simulink model "simulation_X4_PIDout"  (Simulink 8.8)
settings: Solver=ode45  StartTime=0.0  StopTime=10  MaxStep=0.01  RelTol=1e-6  EnableMultiTasking=on
values from neighbouring files (symbols this model uses):
  Ixx = 0.0294853730990492 * 1    (= 0.029485373099)    [main_tune_gain.m]
  Ixz = 0.0000    (= 0)    [main_tune_gain.m]
  Iyy = 0.0636259128602231 * 1    (= 0.0636259128602)    [main_tune_gain.m]
  Izz = 0.0809362287249525 * 1    (= 0.080936228725)    [main_tune_gain.m]
  omega_n_m = 30    [main_tune_gain.m]
  omega_trans_x_out = 0.1    [main_tune_gain.m]
  omega_trans_y_out = 0.1    [main_tune_gain.m]
  omega_trans_z_out = 0.5    [main_tune_gain.m]
  XD = 1.4    [main_tune_gain.m]
  XI = 0.1    [main_tune_gain.m]
  xi_m = 0.707    [main_tune_gain.m]
  XP = 0.1    [main_tune_gain.m]
  YD = 0.4    [main_tune_gain.m]
  YI = 0.1    [main_tune_gain.m]
  YP = 0.8    [main_tune_gain.m]
  ZD = 2    [main_tune_gain.m]
  ZI = 0.02    [main_tune_gain.m]
  ZP = 1    [main_tune_gain.m]
undefined symbols (not defined in the file or in its folder): attitude_control_allocation, compute_com_position
settings Model: SuppressorTable=22 serialization::archive 11 0 3 0 0 0 11 0  Creator=t  LastModifiedBy=root
settings OptimizationCC: ExpressionDepthLimit=2147483647  InitFltsAndDblsToZero=on
settings DebuggingCC: SaveWithParameterizedLinksMsg=none  SolverPrmCheckMsg=warning
settings GRTTargetCC: TargetFcnLib=ansi_tfl_tmw.mat

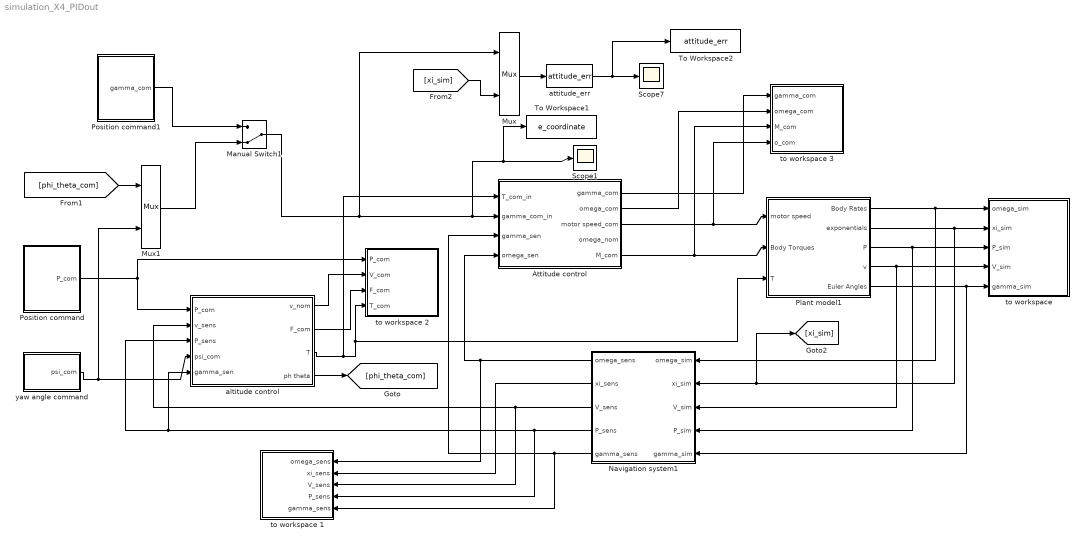
== system simulation_X4_PIDout ==
  Attitude control : Subsystem
  Manual Switch1 : ManualSwitch  CurrentSetting=0
  Mux : Mux  Inputs=2
  Mux1 : Mux  Inputs=2
  Navigation system1 : Subsystem
  Plant model1 : Subsystem
  Position command : Subsystem
  Position command1 : Subsystem
  Scope1 : Scope
  Scope7 : Scope
  To Workspace1 : ToWorkspace  VariableName=e_coordinate  SampleTime=-1
  To Workspace2 : ToWorkspace  VariableName=attitude_err  SampleTime=-1
  altitude control : Subsystem
  attitude_err : MATLABFcn  MATLABFcn=attitude_err
  to workspace : Subsystem
      settings: AttributesFormatString=%<AncestorBlock>
  to workspace 1 : Subsystem
      settings: AttributesFormatString=%<AncestorBlock>
  to workspace 2 : Subsystem
      settings: AttributesFormatString=%<AncestorBlock>
  to workspace 3 : Subsystem
      settings: AttributesFormatString=%<AncestorBlock>
  yaw angle command : Subsystem
  wires:
  Attitude control/3(motor speed_com) -> Plant model1/1(motor speed), to workspace 3/4(o_com)
  Navigation system1/1(omega_sens) -> Attitude control/4(omega_sen), to workspace 1/1(omega_sens)
  Navigation system1/2(xi_sens) -> to workspace 1/2(xi_sens)
  Navigation system1/3(V_sens) -> to workspace 1/3(V_sens), altitude control/2(v_sens)
  Navigation system1/4(P_sens) -> to workspace 1/4(P_sens), altitude control/3(P_sens), altitude control/5(gamma_sen)
  Attitude control/1(gamma_com) -> to workspace 3/1(gamma_com)
  Attitude control/2(omega_com) -> to workspace 3/2(omega_com)
  Attitude control/5(M_com) -> to workspace 3/3(M_com), Plant model1/2(Body Torques)
  Position command/1(P_com) -> altitude control/1(P_com), to workspace 2/1(P_com)
  Plant model1/1(Body Rates) -> to workspace/1(omega_sim), Navigation system1/1(omega_sim)
  Plant model1/2(exponentials) -> to workspace/2(xi_sim), Navigation system1/2(xi_sim), [xi_sim]
  Mux/1 -> attitude_err/1
  attitude_err/1 -> Scope7/1, To Workspace2/1
  altitude control/1(v_nom) -> to workspace 2/2(V_com)
  yaw angle command/1(psi_com) -> Mux1/2, altitude control/4(psi_com)
  Plant model1/3(P) -> to workspace/3(P_sim), Navigation system1/4(P_sim)
  Plant model1/4(v) -> to workspace/4(V_sim), Navigation system1/3(V_sim)
  Plant model1/5(Euler Angles) -> to workspace/5(gamma_sim), Navigation system1/5(gamma_sim)
  Navigation system1/5(gamma_sens) -> to workspace 1/5(gamma_sens), Attitude control/3(gamma_sen)
  [xi_sim] -> Mux/2
  altitude control/2(F_com) -> to workspace 2/3(F_com)
  altitude control/4(ph theta) -> [phi_theta_com]
  [phi_theta_com] -> Mux1/1
  altitude control/3(T) -> Plant model1/3(T), to workspace 2/4(T_com), Attitude control/1(T_com_in)
  Position command1/1(gamma_com) -> Manual Switch1/1
  Manual Switch1/1 -> Attitude control/2(gamma_com_in), Scope1/1, To Workspace1/1, Mux/1
  Mux1/1 -> Manual Switch1/2

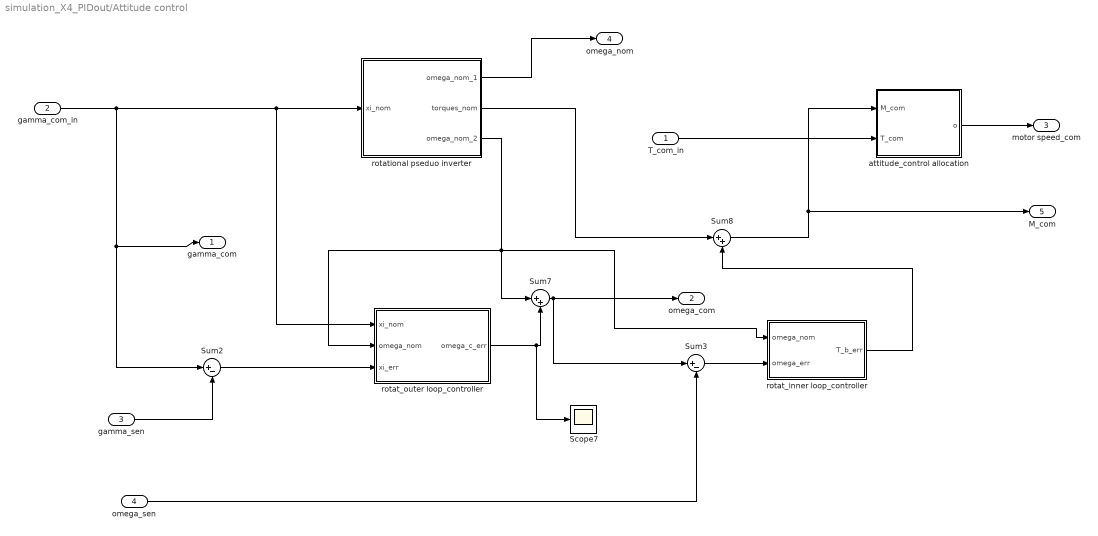
== system simulation_X4_PIDout/Attitude control ==
  T_com_in : Inport
  gamma_com_in : Inport  Port=2
  gamma_sen : Inport  Port=3
  omega_sen : Inport  Port=4
  Scope7 : Scope
  Sum2 : Sum  Inputs=|+-
  Sum3 : Sum  Inputs=|+-
  Sum7 : Sum  Inputs=|++
  Sum8 : Sum  Inputs=|++
  attitude_control allocation : Subsystem
  rotat_inner loop_controller : Subsystem
  rotat_outer loop_controller : Subsystem
  rotational pseduo inverter : Subsystem
  gamma_com : Outport
  omega_com : Outport  Port=2
  motor speed_com : Outport  Port=3
  omega_nom : Outport  Port=4
  M_com : Outport  Port=5
  wires:
  gamma_com_in/1 -> rotational pseduo inverter/1(xi_nom), rotat_outer loop_controller/1(xi_nom), Sum2/1, gamma_com/1
  Sum2/1 -> rotat_outer loop_controller/3(xi_err)
  rotational pseduo inverter/3(omega_nom_2) -> Sum7/1, rotat_outer loop_controller/2(omega_nom), rotat_inner loop_controller/1(omega_nom)
  Sum7/1 -> Sum3/1, omega_com/1
  Sum3/1 -> rotat_inner loop_controller/2(omega_err)
  rotational pseduo inverter/2(torques_nom) -> Sum8/1
  Sum8/1 -> attitude_control allocation/1(M_com), M_com/1
  gamma_sen/1 -> Sum2/2
  omega_sen/1 -> Sum3/2
  rotat_inner loop_controller/1(T_b_err) -> Sum8/2
  rotational pseduo inverter/1(omega_nom_1) -> omega_nom/1
  attitude_control allocation/1(o) -> motor speed_com/1
  T_com_in/1 -> attitude_control allocation/2(T_com)
  rotat_outer loop_controller/1(omega_c_err) -> Sum7/2, Scope7/1

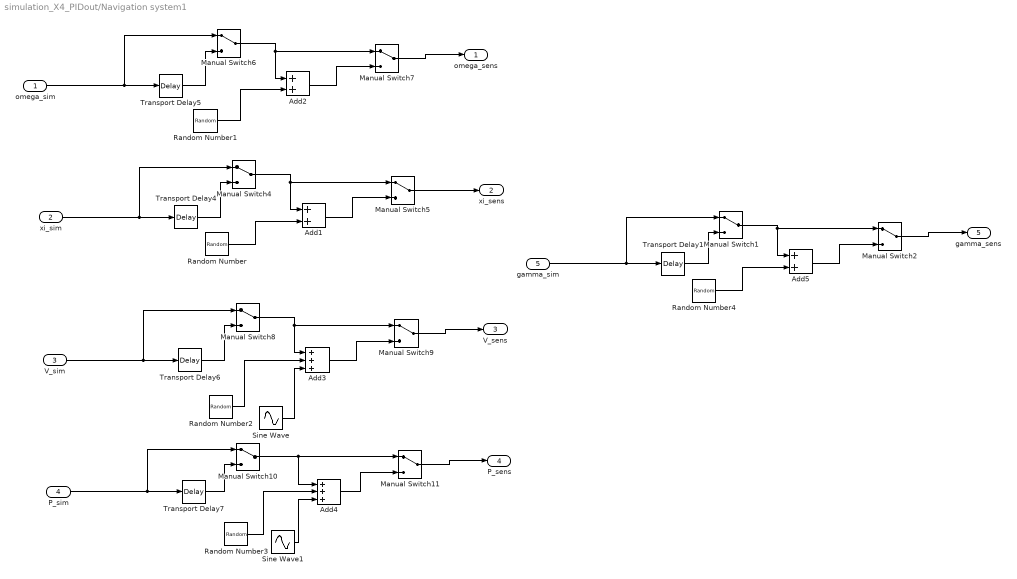
== system simulation_X4_PIDout/Navigation system1 ==
  omega_sim : Inport
  xi_sim : Inport  Port=2
  V_sim : Inport  Port=3
  P_sim : Inport  Port=4
  gamma_sim : Inport  Port=5
  Add1 : Sum
  Add2 : Sum
  Add3 : Sum  Inputs=+++
  Add4 : Sum  Inputs=+++
  Add5 : Sum
  Manual Switch{1..2,4..11} (10 alike) : ManualSwitch
  Random Number : RandomNumber  Variance=0.000025  SampleTime=0
  Random Number1 : RandomNumber  Variance=0.001  SampleTime=0
  Random Number2 : RandomNumber  Variance=0.001  SampleTime=0
  Random Number3 : RandomNumber  Variance=0.001  SampleTime=0
  Random Number4 : RandomNumber  Variance=0.000025  SampleTime=0
  Sine Wave : Sin  Amplitude=0.2  SampleTime=0
  Sine Wave1 : Sin  Amplitude=1.5  SampleTime=0
  Transport Delay1 : TransportDelay  DelayTime=0.02
  Transport Delay4 : TransportDelay  DelayTime=0.02
  Transport Delay5 : TransportDelay  DelayTime=0.02
  Transport Delay6 : TransportDelay  DelayTime=0.4
  Transport Delay7 : TransportDelay  DelayTime=0.4
  omega_sens : Outport
  xi_sens : Outport  Port=2
  V_sens : Outport  Port=3
  P_sens : Outport  Port=4
  gamma_sens : Outport  Port=5
  wires:
  xi_sim/1 -> Transport Delay4/1, Manual Switch4/1
  Manual Switch4/1 -> Add1/1, Manual Switch5/1
  Transport Delay4/1 -> Manual Switch4/2
  Manual Switch5/1 -> xi_sens/1
  Random Number/1 -> Add1/2
  Add1/1 -> Manual Switch5/2
  omega_sim/1 -> Transport Delay5/1, Manual Switch6/1
  Manual Switch6/1 -> Add2/1, Manual Switch7/1
  Transport Delay5/1 -> Manual Switch6/2
  Manual Switch7/1 -> omega_sens/1
  Random Number1/1 -> Add2/2
  Add2/1 -> Manual Switch7/2
  V_sim/1 -> Transport Delay6/1, Manual Switch8/1
  Manual Switch8/1 -> Add3/1, Manual Switch9/1
  Transport Delay6/1 -> Manual Switch8/2
  Manual Switch9/1 -> V_sens/1
  Random Number2/1 -> Add3/2
  Add3/1 -> Manual Switch9/2
  P_sim/1 -> Transport Delay7/1, Manual Switch10/1
  Manual Switch10/1 -> Add4/1, Manual Switch11/1
  Transport Delay7/1 -> Manual Switch10/2
  Manual Switch11/1 -> P_sens/1
  Random Number3/1 -> Add4/2
  Add4/1 -> Manual Switch11/2
  gamma_sim/1 -> Transport Delay1/1, Manual Switch1/1
  Manual Switch1/1 -> Add5/1, Manual Switch2/1
  Transport Delay1/1 -> Manual Switch1/2
  Manual Switch2/1 -> gamma_sens/1
  Random Number4/1 -> Add5/2
  Add5/1 -> Manual Switch2/2
  Sine Wave/1 -> Add3/3
  Sine Wave1/1 -> Add4/3

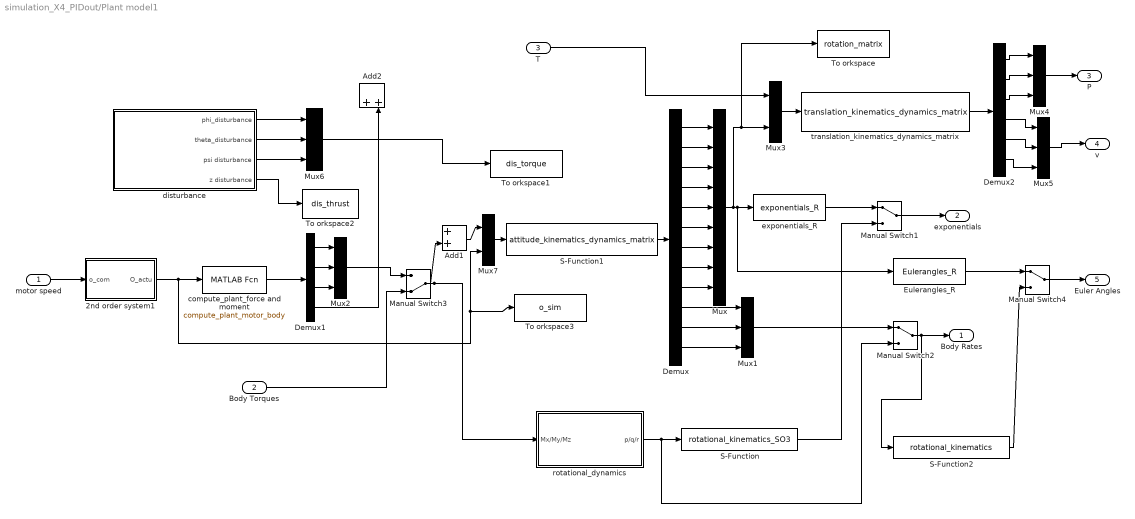
== system simulation_X4_PIDout/Plant model1 ==
  motor speed : Inport
  Body Torques : Inport  Port=2
  T : Inport  Port=3
  2nd order system1 : Subsystem
  Add1 : Sum
  Add2 : Sum
  Demux : Demux  Outputs=12
  Demux1 : Demux
  Demux2 : Demux  Outputs=6
  Eulerangles_R : MATLABFcn  MATLABFcn=Eulerangles_R  OutputDimensions=3
  Manual Switch1 : ManualSwitch
  Manual Switch2 : ManualSwitch
  Manual Switch3 : ManualSwitch  CurrentSetting=0
  Manual Switch4 : ManualSwitch
  Mux : Mux  Inputs=9
  Mux{1..2,4..6} (5 alike) : Mux  Inputs=3
  Mux3 : Mux  Inputs=2
  Mux7 : Mux  Inputs=2
  S-Function : S-Function  FunctionName=rotational_kinematics_SO3  SFunctionDeploymentMode=off  EnableBusSupport=off
  S-Function1 : S-Function  FunctionName=attitude_kinematics_dynamics_matrix  SFunctionDeploymentMode=off  EnableBusSupport=off
  S-Function2 : S-Function  FunctionName=rotational_kinematics  SFunctionDeploymentMode=off  EnableBusSupport=off
  To orkspace : ToWorkspace  VariableName=rotation_matrix  SampleTime=-1
  To orkspace1 : ToWorkspace  VariableName=dis_torque  SampleTime=-1
  To orkspace2 : ToWorkspace  VariableName=dis_thrust  SampleTime=-1
  To orkspace3 : ToWorkspace  VariableName=o_sim  SampleTime=-1
  compute_plant_force and moment : MATLABFcn  MATLABFcn=compute_plant_motor_body
  disturbance : Subsystem
  exponentials_R : MATLABFcn  MATLABFcn=exponentials_R  OutputDimensions=3
  rotational_dynamics : Subsystem
  translation_kinematics_dynamics_matrix : S-Function  FunctionName=translation_kinematics_dynamics_matrix  SFunctionDeploymentMode=off  EnableBusSupport=off
  Body Rates : Outport
  exponentials : Outport  Port=2
  P : Outport  Port=3
  v : Outport  Port=4
  Euler Angles : Outport  Port=5
  wires:
  rotational_dynamics/1(p/q/r) -> S-Function/1, Manual Switch2/2
  S-Function1/1 -> Demux/1
  Demux/1 -> Mux/1
  Demux/2 -> Mux/2
  Demux/3 -> Mux/3
  Demux/4 -> Mux/4
  Demux/5 -> Mux/5
  Demux/6 -> Mux/6
  Demux/7 -> Mux/7
  Demux/8 -> Mux/8
  Demux/9 -> Mux/9
  Demux/10 -> Mux1/1
  Demux/11 -> Mux1/2
  Demux/12 -> Mux1/3
  Mux/1 -> exponentials_R/1, Eulerangles_R/1, Mux3/2, To orkspace/1
  exponentials_R/1 -> Manual Switch1/1
  Mux1/1 -> Manual Switch2/1
  S-Function/1 -> Manual Switch1/2
  Manual Switch1/1 -> exponentials/1
  Manual Switch2/1 -> Body Rates/1, S-Function2/1
  motor speed/1 -> 2nd order system1/1(o_com)
  compute_plant_force and moment/1 -> Demux1/1
  Demux1/1 -> Mux2/1
  Demux1/2 -> Mux2/2
  Demux1/3 -> Mux2/3
  Mux2/1 -> Manual Switch3/1
  Manual Switch3/1 -> rotational_dynamics/1(Mx/My/Mz), Add1/2
  Body Torques/1 -> Manual Switch3/2
  Mux3/1 -> translation_kinematics_dynamics_matrix/1
  translation_kinematics_dynamics_matrix/1 -> Demux2/1
  Demux2/1 -> Mux4/1
  Demux2/2 -> Mux4/2
  Demux2/3 -> Mux4/3
  Demux2/4 -> Mux5/1
  Demux2/5 -> Mux5/2
  Demux2/6 -> Mux5/3
  Mux4/1 -> P/1
  Mux5/1 -> v/1
  Eulerangles_R/1 -> Manual Switch4/1
  S-Function2/1 -> Manual Switch4/2
  Manual Switch4/1 -> Euler Angles/1
  disturbance/1(phi_disturbance) -> Mux6/1
  disturbance/2(theta_disturbance) -> Mux6/2
  disturbance/3(psi disturbance) -> Mux6/3
  Mux6/1 -> To orkspace1/1
  disturbance/4(z disturbance) -> To orkspace2/1
  Demux1/4 -> Add2/2
  2nd order system1/1(O_actu) -> compute_plant_force and moment/1, Mux7/2, To orkspace3/1
  Mux7/1 -> S-Function1/1
  Add1/1 -> Mux7/1
  T/1 -> Mux3/1

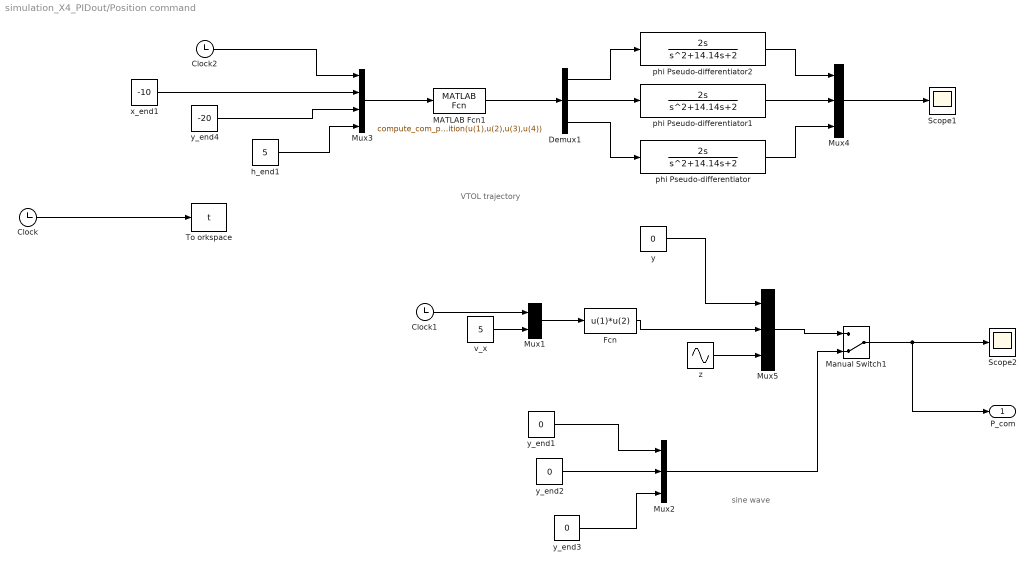
== system simulation_X4_PIDout/Position command ==
  note: VTOL trajectory
  note: sine wave
  Clock : Clock
  Clock1 : Clock
  Clock2 : Clock
  Demux1 : Demux  Outputs=3
  Fcn : Fcn  Expr=u(1)*u(2)
  MATLAB Fcn1 : MATLABFcn  MATLABFcn=compute_com_position(u(1),u(2),u(3),u(4))
  Manual Switch1 : ManualSwitch  CurrentSetting=0
  Mux1 : Mux  Inputs=2
  Mux2 : Mux  Inputs=3
  Mux3 : Mux
  Mux4 : Mux  Inputs=3
  Mux5 : Mux  Inputs=3
  Scope1 : Scope
  Scope2 : Scope
  To orkspace : ToWorkspace  VariableName=t  SampleTime=-1
  h_end1 : Constant  Value=5
  phi Pseudo-differentiator : TransferFcn  Numerator=[2 0]  Denominator=[1 14.14 2]
  phi Pseudo-differentiator1 : TransferFcn  Numerator=[2 0]  Denominator=[1 14.14 2]
  phi Pseudo-differentiator2 : TransferFcn  Numerator=[2 0]  Denominator=[1 14.14 2]
  v_x : Constant  Value=5
  x_end1 : Constant  Value=-10
  y : Constant  Value=0
  y_end1 : Constant  Value=0
  y_end2 : Constant  Value=0
  y_end3 : Constant  Value=0
  y_end4 : Constant  Value=-20
  z : Sin  Frequency=0.5  SampleTime=0
  P_com : Outport
  wires:
  y_end1/1 -> Mux2/1
  y_end2/1 -> Mux2/2
  y_end3/1 -> Mux2/3
  Mux3/1 -> MATLAB Fcn1/1
  Clock2/1 -> Mux3/1
  x_end1/1 -> Mux3/2
  y_end4/1 -> Mux3/3
  h_end1/1 -> Mux3/4
  Demux1/1 -> phi Pseudo-differentiator2/1
  Demux1/2 -> phi Pseudo-differentiator1/1
  Demux1/3 -> phi Pseudo-differentiator/1
  phi Pseudo-differentiator2/1 -> Mux4/1
  phi Pseudo-differentiator1/1 -> Mux4/2
  phi Pseudo-differentiator/1 -> Mux4/3
  MATLAB Fcn1/1 -> Demux1/1
  Mux4/1 -> Scope1/1
  Mux1/1 -> Fcn/1
  Clock1/1 -> Mux1/1
  v_x/1 -> Mux1/2
  Fcn/1 -> Mux5/2
  y/1 -> Mux5/1
  z/1 -> Mux5/3
  Clock/1 -> To orkspace/1
  Mux5/1 -> Manual Switch1/1
  Manual Switch1/1 -> Scope2/1, P_com/1
  Mux2/1 -> Manual Switch1/2

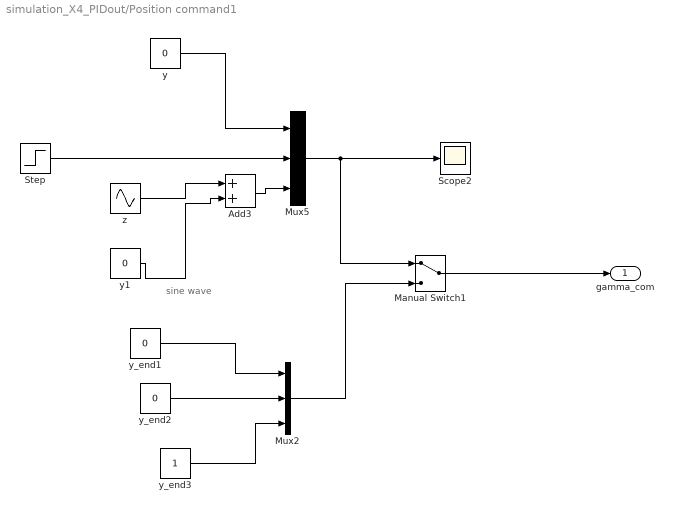
== system simulation_X4_PIDout/Position command1 ==
  note: sine wave
  Add3 : Sum
  Manual Switch1 : ManualSwitch
  Mux2 : Mux  Inputs=3
  Mux5 : Mux  Inputs=3
  Scope2 : Scope
  Step : Step  Time=2  After=0.1  SampleTime=0
  y : Constant  Value=0
  y1 : Constant  Value=0
  y_end1 : Constant  Value=0
  y_end2 : Constant  Value=0
  y_end3 : Constant
  z : Sin  Amplitude=0.1  Frequency=0.5  SampleTime=0
  gamma_com : Outport
  wires:
  y_end1/1 -> Mux2/1
  y_end2/1 -> Mux2/2
  y_end3/1 -> Mux2/3
  Mux5/1 -> Scope2/1, Manual Switch1/1
  y/1 -> Mux5/1
  Mux2/1 -> Manual Switch1/2
  Manual Switch1/1 -> gamma_com/1
  Step/1 -> Mux5/2
  z/1 -> Add3/1
  Add3/1 -> Mux5/3
  y1/1 -> Add3/2

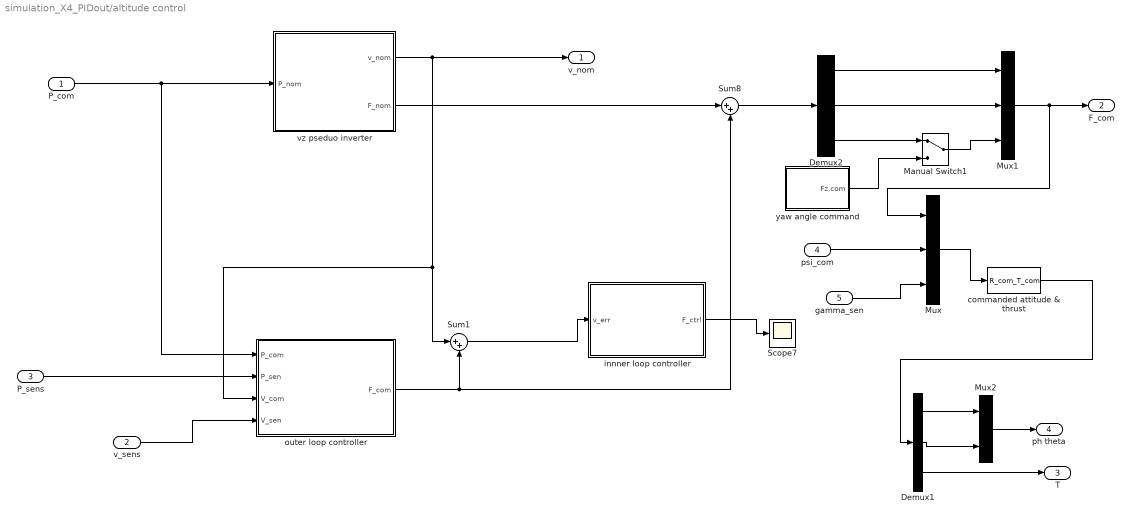
== system simulation_X4_PIDout/altitude control ==
  P_com : Inport
  v_sens : Inport  Port=2
  P_sens : Inport  Port=3
  psi_com : Inport  Port=4
  gamma_sen : Inport  Port=5
  Demux1 : Demux  Outputs=3
  Demux2 : Demux  Outputs=3
  Manual Switch1 : ManualSwitch
  Mux : Mux  Inputs=3
  Mux1 : Mux  Inputs=3
  Mux2 : Mux  Inputs=2
  Scope7 : Scope
  Sum1 : Sum  Inputs=|++
  Sum8 : Sum  Inputs=|++
  commanded attitude & thrust : MATLABFcn  MATLABFcn=R_com_T_com
  innner loop controller : Subsystem
  outer loop controller : Subsystem
  vz pseduo inverter : Subsystem
  yaw angle command : Subsystem
  v_nom : Outport
  F_com : Outport  Port=2
  T : Outport  Port=3
  ph theta : Outport  Port=4
  wires:
  P_com/1 -> vz pseduo inverter/1(P_nom), outer loop controller/1(P_com)
  innner loop controller/1(F_ctrl) -> Scope7/1
  vz pseduo inverter/2(F_nom) -> Sum8/1
  P_sens/1 -> outer loop controller/2(P_sen)
  vz pseduo inverter/1(v_nom) -> v_nom/1, Sum1/1, outer loop controller/3(V_com)
  outer loop controller/1(F_com) -> Sum1/2, Sum8/2
  Sum1/1 -> innner loop controller/1(v_err)
  psi_com/1 -> Mux/2
  Mux/1 -> commanded attitude & thrust/1
  Demux1/1 -> Mux2/1
  Demux1/2 -> Mux2/2
  commanded attitude & thrust/1 -> Demux1/1
  Mux2/1 -> ph theta/1
  Demux1/3 -> T/1
  Sum8/1 -> Demux2/1
  Demux2/3 -> Manual Switch1/1
  Demux2/1 -> Mux1/1
  Demux2/2 -> Mux1/2
  Manual Switch1/1 -> Mux1/3
  Mux1/1 -> F_com/1, Mux/1
  yaw angle command/1(Fz,com) -> Manual Switch1/2
  v_sens/1 -> outer loop controller/4(V_sen)
  gamma_sen/1 -> Mux/3

== system simulation_X4_PIDout/to workspace ==
  omega_sim : Inport
  xi_sim : Inport  Port=2
  P_sim : Inport  Port=3
  V_sim : Inport  Port=4
  gamma_sim : Inport  Port=5
  To Workspace1 : ToWorkspace  VariableName=gamma_sim  SampleTime=-1
  To Workspace2 : ToWorkspace  VariableName=V_sim  SampleTime=-1
  To Workspace3 : ToWorkspace  VariableName=P_sim  SampleTime=-1
  To Workspace4 : ToWorkspace  VariableName=xi_sim  SampleTime=-1
  To orkspace : ToWorkspace  VariableName=omega_sim  SampleTime=-1
  wires:
  omega_sim/1 -> To orkspace/1
  V_sim/1 -> To Workspace2/1
  P_sim/1 -> To Workspace3/1
  gamma_sim/1 -> To Workspace1/1
  xi_sim/1 -> To Workspace4/1

== system simulation_X4_PIDout/to workspace 1 ==
  omega_sens : Inport
  xi_sens : Inport  Port=2
  V_sens : Inport  Port=3
  P_sens : Inport  Port=4
  gamma_sens : Inport  Port=5
  To Workspace1 : ToWorkspace  VariableName=gamma_sens  SampleTime=-1
  To Workspace2 : ToWorkspace  VariableName=V_sens  SampleTime=-1
  To Workspace3 : ToWorkspace  VariableName=P_sens  SampleTime=-1
  To Workspace4 : ToWorkspace  VariableName=xi_sens  SampleTime=-1
  To orkspace : ToWorkspace  VariableName=omega_sens  SampleTime=-1
  wires:
  omega_sens/1 -> To orkspace/1
  xi_sens/1 -> To Workspace4/1
  V_sens/1 -> To Workspace2/1
  P_sens/1 -> To Workspace3/1
  gamma_sens/1 -> To Workspace1/1

== system simulation_X4_PIDout/to workspace 2 ==
  P_com : Inport
  V_com : Inport  Port=2
  F_com : Inport  Port=3
  T_com : Inport  Port=4
  To Workspace1 : ToWorkspace  VariableName=V_com  SampleTime=-1
  To Workspace2 : ToWorkspace  VariableName=F_com  SampleTime=-1
  To Workspace3 : ToWorkspace  VariableName=T_com  SampleTime=-1
  To orkspace : ToWorkspace  VariableName=P_com  SampleTime=-1
  wires:
  P_com/1 -> To orkspace/1
  V_com/1 -> To Workspace1/1
  F_com/1 -> To Workspace2/1
  T_com/1 -> To Workspace3/1

== system simulation_X4_PIDout/to workspace 3 ==
  gamma_com : Inport
  omega_com : Inport  Port=2
  M_com : Inport  Port=3
  o_com : Inport  Port=4
  To Workspace1 : ToWorkspace  VariableName=omega_com  SampleTime=-1
  To Workspace2 : ToWorkspace  VariableName=M_com  SampleTime=-1
  To Workspace3 : ToWorkspace  VariableName=o_com  SampleTime=-1
  To Workspace4 : ToWorkspace  VariableName=gamma_com  SampleTime=-1
  wires:
  gamma_com/1 -> To Workspace4/1
  omega_com/1 -> To Workspace1/1
  M_com/1 -> To Workspace2/1
  o_com/1 -> To Workspace3/1

== system simulation_X4_PIDout/yaw angle command ==
  note: sine wave
  Manual Switch5 : ManualSwitch  CurrentSetting=0
  y_end1 : Constant  Value=0
  z : Sin  Frequency=0.5  SampleTime=0
  psi_com : Outport
  wires:
  z/1 -> Manual Switch5/1
  y_end1/1 -> Manual Switch5/2
  Manual Switch5/1 -> psi_com/1

== system simulation_X4_PIDout/Attitude control/attitude_control allocation ==
  M_com : Inport
  T_com : Inport  Port=2
  MATLAB Fcn : MATLABFcn  MATLABFcn=attitude_control_allocation(u(1),u(2),u(3),u(4))
  Mux : Mux  Inputs=2
  o : Outport
  wires:
  T_com/1 -> Mux/2
  Mux/1 -> MATLAB Fcn/1
  MATLAB Fcn/1 -> o/1
  M_com/1 -> Mux/1

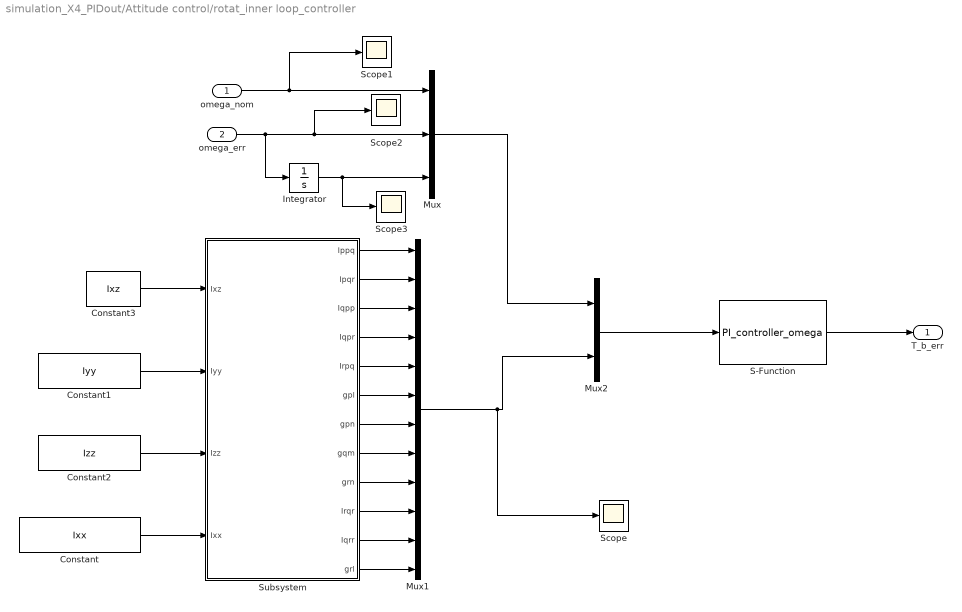
== system simulation_X4_PIDout/Attitude control/rotat_inner loop_controller ==
  omega_nom : Inport
  omega_err : Inport  Port=2
  Constant : Constant  Value=Ixx
  Constant1 : Constant  Value=Iyy
  Constant2 : Constant  Value=Izz
  Constant3 : Constant  Value=Ixz
  Integrator : Integrator
  Mux : Mux  Inputs=3
  Mux1 : Mux  Inputs=12
  Mux2 : Mux  Inputs=2
  S-Function : S-Function  FunctionName=PI_controller_omega  SFunctionDeploymentMode=off  EnableBusSupport=off
  Scope{,1..3} (4 alike) : Scope
  Subsystem : Subsystem
  T_b_err : Outport
  wires:
  omega_err/1 -> Integrator/1, Mux/2, Scope2/1
  omega_nom/1 -> Mux/1, Scope1/1
  Integrator/1 -> Mux/3, Scope3/1
  Subsystem/1(Ippq) -> Mux1/1
  Subsystem/2(Ipqr) -> Mux1/2
  Subsystem/3(Iqpp) -> Mux1/3
  Subsystem/4(Iqpr) -> Mux1/4
  Subsystem/5(Irpq) -> Mux1/5
  Subsystem/6(gpl) -> Mux1/6
  Subsystem/7(gpn) -> Mux1/7
  Subsystem/8(gqm) -> Mux1/8
  Subsystem/9(grn) -> Mux1/9
  Subsystem/10(Irqr) -> Mux1/10
  Subsystem/11(Iqrr) -> Mux1/11
  Subsystem/12(grl) -> Mux1/12
  Mux/1 -> Mux2/1
  Mux1/1 -> Mux2/2, Scope/1
  Mux2/1 -> S-Function/1
  S-Function/1 -> T_b_err/1
  Constant2/1 -> Subsystem/3(Izz)
  Constant/1 -> Subsystem/4(Ixx)
  Constant1/1 -> Subsystem/2(Iyy)
  Constant3/1 -> Subsystem/1(Ixz)

== system simulation_X4_PIDout/Attitude control/rotat_outer loop_controller ==
  xi_nom : Inport
  omega_nom : Inport  Port=2
  xi_err : Inport  Port=3
  Integrator : Integrator
  Mux : Mux
  S-Function : S-Function  FunctionName=PI_controller_gamma  SFunctionDeploymentMode=off  EnableBusSupport=off
  Scope{,1..4} (5 alike) : Scope
  omega_c_err : Outport
  wires:
  xi_err/1 -> Integrator/1, Mux/3, Scope3/1
  Integrator/1 -> Mux/4, Scope1/1
  omega_nom/1 -> Mux/2, Scope4/1
  xi_nom/1 -> Mux/1, Scope2/1
  Mux/1 -> S-Function/1
  S-Function/1 -> omega_c_err/1, Scope/1

== system simulation_X4_PIDout/Attitude control/rotational pseduo inverter ==
  xi_nom : Inport
  Mux7 : Mux  Inputs=2
  Mux9 : Mux  Inputs=2
  S-Function3 : S-Function  FunctionName=omega_nom  SFunctionDeploymentMode=off  EnableBusSupport=off
  S-Function4 : S-Function  FunctionName=torque_nom  SFunctionDeploymentMode=off  EnableBusSupport=off
  pseudodifferentiator : Subsystem
  pseudodifferentiator1 : Subsystem
  omega_nom_1 : Outport
  torques_nom : Outport  Port=2
  omega_nom_2 : Outport  Port=3
  wires:
  xi_nom/1 -> Mux7/1, pseudodifferentiator/1(In1)
  Mux7/1 -> S-Function3/1
  S-Function3/1 -> pseudodifferentiator1/1(In1), Mux9/1, omega_nom_1/1, omega_nom_2/1
  Mux9/1 -> S-Function4/1
  S-Function4/1 -> torques_nom/1
  pseudodifferentiator/1(Out1) -> Mux7/2
  pseudodifferentiator1/1(Out1) -> Mux9/2

== system simulation_X4_PIDout/Plant model1/2nd order system1 ==
  o_com : Inport
  2order : Subsystem
  2order1 : Subsystem
  2order2 : Subsystem
  2order3 : Subsystem
  Demux : Demux
  Manual Switch3 : ManualSwitch
  Mux : Mux
  O_actu : Outport
  wires:
  Demux/2 -> 2order1/1(In1)
  2order2/1(Out1) -> Mux/3
  Demux/3 -> 2order2/1(In1)
  2order1/1(Out1) -> Mux/2
  o_com/1 -> Demux/1, Manual Switch3/1
  Demux/4 -> 2order3/1(In1)
  2order3/1(Out1) -> Mux/4
  Demux/1 -> 2order/1(In1)
  2order/1(Out1) -> Mux/1
  Mux/1 -> Manual Switch3/2
  Manual Switch3/1 -> O_actu/1

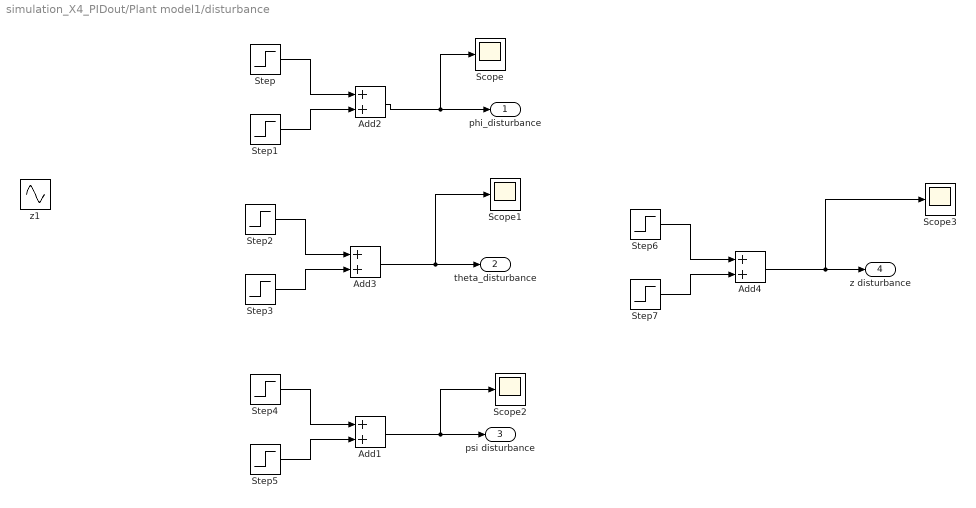
== system simulation_X4_PIDout/Plant model1/disturbance ==
  Add{1..4} (4 alike) : Sum
  Scope{,1..3} (4 alike) : Scope
  Step : Step  Time=5  After=0.3  SampleTime=0
  Step1 : Step  Time=6  After=-0.3  SampleTime=0
  Step2 : Step  Time=9  After=0.3  SampleTime=0
  Step3 : Step  Time=10  After=-0.3  SampleTime=0
  Step4 : Step  Time=13  After=0.1  SampleTime=0
  Step5 : Step  Time=14  After=-0.1  SampleTime=0
  Step6 : Step  Time=16  After=-10  SampleTime=0
  Step7 : Step  Time=17  After=10  SampleTime=0
  z1 : Sin  Amplitude=0.1  Frequency=3*pi  SampleTime=0
  phi_disturbance : Outport
  theta_disturbance : Outport  Port=2
  psi disturbance : Outport  Port=3
  z disturbance : Outport  Port=4
  wires:
  Step/1 -> Add2/1
  Step1/1 -> Add2/2
  Step2/1 -> Add3/1
  Step3/1 -> Add3/2
  Add2/1 -> phi_disturbance/1, Scope/1
  Add3/1 -> theta_disturbance/1, Scope1/1
  Step4/1 -> Add1/1
  Step5/1 -> Add1/2
  Add1/1 -> psi disturbance/1, Scope2/1
  Step6/1 -> Add4/1
  Step7/1 -> Add4/2
  Add4/1 -> z disturbance/1, Scope3/1

== system simulation_X4_PIDout/Plant model1/rotational_dynamics ==
  Mx/My/Mz : Inport
  Constant : Constant  Value=0.010914387
  Constant1 : Constant  Value=0.011174571
  Constant2 : Constant  Value=0.020874735
  Constant3 : Constant  Value=0
  Mux : Mux  Inputs=13
  S-Function : S-Function  FunctionName=rotational_dynamics  SFunctionDeploymentMode=off  EnableBusSupport=off
  Subsystem1 : Subsystem
  p/q/r : Outport
  wires:
  Constant2/1 -> Subsystem1/3(Izz)
  Constant/1 -> Subsystem1/4(Ixx)
  Constant1/1 -> Subsystem1/2(Iyy)
  Constant3/1 -> Subsystem1/1(Ixz)
  Mx/My/Mz/1 -> Mux/1
  Subsystem1/1(Ippq) -> Mux/2
  Subsystem1/2(Ipqr) -> Mux/3
  Subsystem1/3(Iqpp) -> Mux/4
  Subsystem1/4(Iqpr) -> Mux/5
  Subsystem1/5(Irpq) -> Mux/6
  Subsystem1/6(gpl) -> Mux/7
  Subsystem1/7(gpn) -> Mux/8
  Subsystem1/8(gqm) -> Mux/9
  Subsystem1/9(grn) -> Mux/10
  Subsystem1/10(Irqr) -> Mux/11
  Subsystem1/11(Iqrr) -> Mux/12
  Subsystem1/12(grl) -> Mux/13
  Mux/1 -> S-Function/1
  S-Function/1 -> p/q/r/1

== system simulation_X4_PIDout/altitude control/innner loop controller ==
  v_err : Inport
  Demux : Demux  Outputs=3
  Mux : Mux  Inputs=3
  Scope1 : Scope
  Subsystem : Subsystem
  Subsystem1 : Subsystem
  Subsystem2 : Subsystem
  F_ctrl : Outport
  wires:
  v_err/1 -> Demux/1
  Demux/1 -> Subsystem/1(In1)
  Demux/2 -> Subsystem1/1(In1)
  Demux/3 -> Subsystem2/1(In1)
  Subsystem/1(Out1) -> Mux/1
  Subsystem1/1(Out1) -> Mux/2
  Subsystem2/1(Out1) -> Mux/3
  Mux/1 -> F_ctrl/1, Scope1/1

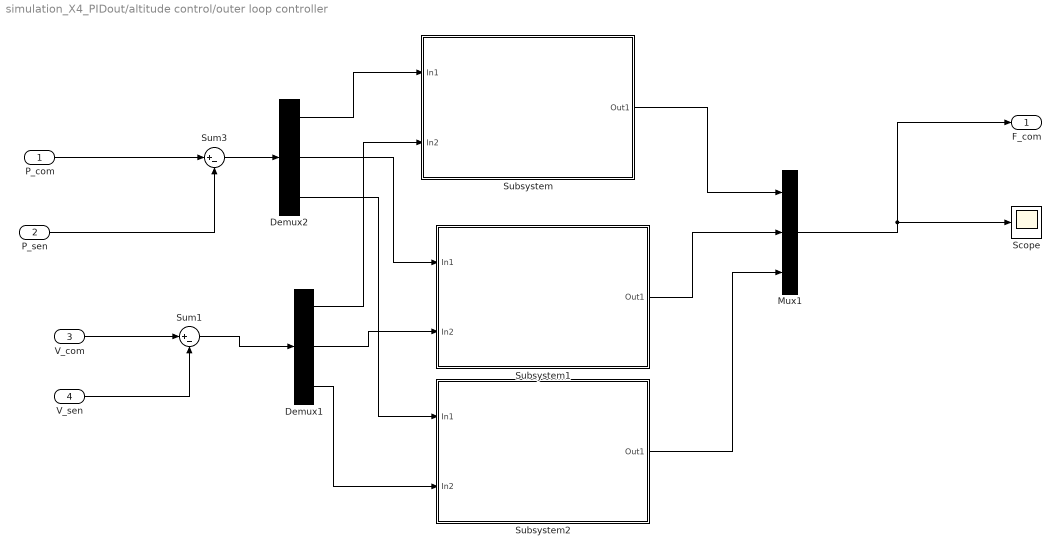
== system simulation_X4_PIDout/altitude control/outer loop controller ==
  P_com : Inport
  P_sen : Inport  Port=2
  V_com : Inport  Port=3
  V_sen : Inport  Port=4
  Demux1 : Demux  Outputs=3
  Demux2 : Demux  Outputs=3
  Mux1 : Mux  Inputs=3
  Scope : Scope
  Subsystem : Subsystem
  Subsystem1 : Subsystem
  Subsystem2 : Subsystem
  Sum1 : Sum  Inputs=|+-
  Sum3 : Sum  Inputs=|+-
  F_com : Outport
  wires:
  P_sen/1 -> Sum3/2
  P_com/1 -> Sum3/1
  V_com/1 -> Sum1/1
  V_sen/1 -> Sum1/2
  Sum3/1 -> Demux2/1
  Sum1/1 -> Demux1/1
  Demux2/1 -> Subsystem/1(In1)
  Demux1/1 -> Subsystem/2(In2)
  Demux2/2 -> Subsystem1/1(In1)
  Demux1/2 -> Subsystem1/2(In2)
  Demux2/3 -> Subsystem2/1(In1)
  Demux1/3 -> Subsystem2/2(In2)
  Subsystem/1(Out1) -> Mux1/1
  Subsystem1/1(Out1) -> Mux1/2
  Subsystem2/1(Out1) -> Mux1/3
  Mux1/1 -> F_com/1, Scope/1

== system simulation_X4_PIDout/altitude control/vz pseduo inverter ==
  P_nom : Inport
  mass : Gain  Gain=0.975
  pseudodifferentiator : Subsystem
  pseudodifferentiator1 : Subsystem
  v_nom : Outport
  F_nom : Outport  Port=2
  wires:
  P_nom/1 -> pseudodifferentiator/1(In1)
  pseudodifferentiator/1(Out1) -> v_nom/1, pseudodifferentiator1/1(In1)
  pseudodifferentiator1/1(Out1) -> mass/1
  mass/1 -> F_nom/1

== system simulation_X4_PIDout/altitude control/yaw angle command ==
  note: sine wave
  Manual Switch5 : ManualSwitch
  y_end1 : Constant  Value=0
  z : Sin  Amplitude=10  Frequency=0.5  SampleTime=0
  Fz,com : Outport
  wires:
  z/1 -> Manual Switch5/1
  y_end1/1 -> Manual Switch5/2
  Manual Switch5/1 -> Fz,com/1

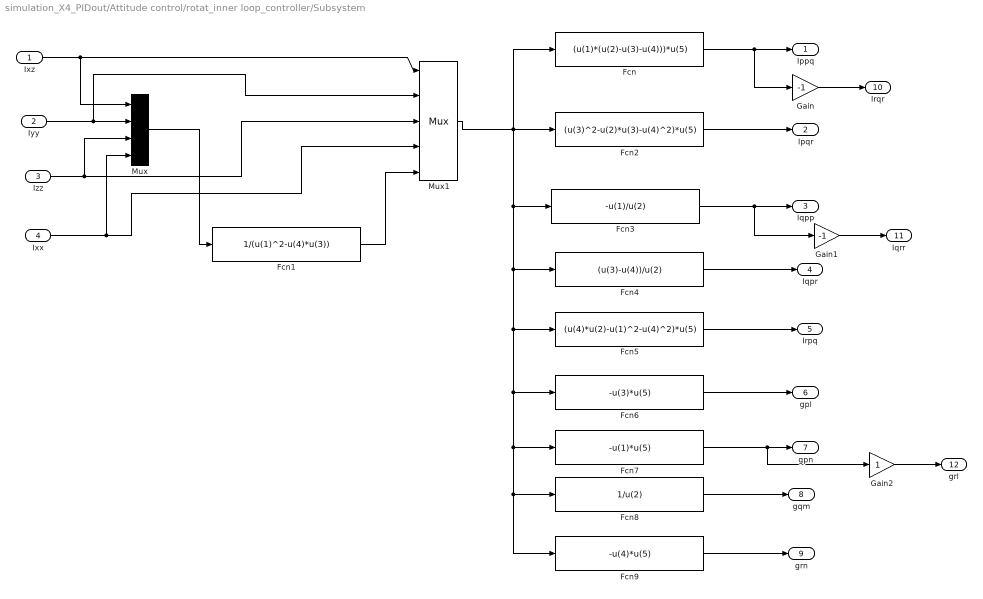
== system simulation_X4_PIDout/Attitude control/rotat_inner loop_controller/Subsystem ==
  Ixz : Inport
  Iyy : Inport  Port=2
  Izz : Inport  Port=3
  Ixx : Inport  Port=4
  Fcn : Fcn  Expr=(u(1)*(u(2)-u(3)-u(4)))*u(5)
  Fcn1 : Fcn  Expr=1/(u(1)^2-u(4)*u(3))
  Fcn2 : Fcn  Expr=(u(3)^2-u(2)*u(3)-u(4)^2)*u(5)
  Fcn3 : Fcn  Expr=-u(1)/u(2)
  Fcn4 : Fcn  Expr=(u(3)-u(4))/u(2)
  Fcn5 : Fcn  Expr=(u(4)*u(2)-u(1)^2-u(4)^2)*u(5)
  Fcn6 : Fcn  Expr=-u(3)*u(5)
  Fcn7 : Fcn  Expr=-u(1)*u(5)
  Fcn8 : Fcn  Expr=1/u(2)
  Fcn9 : Fcn  Expr=-u(4)*u(5)
  Gain : Gain  Gain=-1
  Gain1 : Gain  Gain=-1
  Gain2 : Gain
  Mux : Mux
  Mux1 : Mux  Inputs=5
  Ippq : Outport
  Ipqr : Outport  Port=2
  Iqpp : Outport  Port=3
  Iqpr : Outport  Port=4
  Irpq : Outport  Port=5
  gpl : Outport  Port=6
  gpn : Outport  Port=7
  gqm : Outport  Port=8
  grn : Outport  Port=9
  Irqr : Outport  Port=10
  Iqrr : Outport  Port=11
  grl : Outport  Port=12
  wires:
  Ixz/1 -> Mux/1, Mux1/1
  Iyy/1 -> Mux/2, Mux1/2
  Izz/1 -> Mux/3, Mux1/3
  Ixx/1 -> Mux/4, Mux1/4
  Mux/1 -> Fcn1/1
  Fcn1/1 -> Mux1/5
  Fcn/1 -> Ippq/1, Gain/1
  Mux1/1 -> Fcn/1, Fcn2/1, Fcn3/1, Fcn4/1, Fcn5/1, Fcn6/1, Fcn7/1, Fcn8/1, Fcn9/1
  Fcn2/1 -> Ipqr/1
  Fcn3/1 -> Iqpp/1, Gain1/1
  Fcn4/1 -> Iqpr/1
  Fcn5/1 -> Irpq/1
  Fcn6/1 -> gpl/1
  Fcn7/1 -> gpn/1, Gain2/1
  Fcn8/1 -> gqm/1
  Fcn9/1 -> grn/1
  Gain/1 -> Irqr/1
  Gain1/1 -> Iqrr/1
  Gain2/1 -> grl/1

== system simulation_X4_PIDout/Attitude control/rotational pseduo inverter/pseudodifferentiator ==
  In1 : Inport
  Demux : Demux  Outputs=3
  Mux : Mux  Inputs=3
  pseudodifferentiator1 : Subsystem
  pseudodifferentiator2 : Subsystem
  pseudodifferentiator3 : Subsystem
  Out1 : Outport
  wires:
  Demux/1 -> pseudodifferentiator2/1(In1)
  Demux/2 -> pseudodifferentiator1/1(In1)
  Demux/3 -> pseudodifferentiator3/1(In1)
  pseudodifferentiator3/1(Out1) -> Mux/3
  pseudodifferentiator1/1(Out1) -> Mux/2
  pseudodifferentiator2/1(Out1) -> Mux/1
  In1/1 -> Demux/1
  Mux/1 -> Out1/1

== system simulation_X4_PIDout/Attitude control/rotational pseduo inverter/pseudodifferentiator1 ==
  In1 : Inport
  Demux : Demux  Outputs=3
  Mux : Mux  Inputs=3
  pseudodifferentiator1 : Subsystem
  pseudodifferentiator2 : Subsystem
  pseudodifferentiator3 : Subsystem
  Out1 : Outport
  wires:
  Demux/1 -> pseudodifferentiator2/1(In1)
  Demux/2 -> pseudodifferentiator1/1(In1)
  Demux/3 -> pseudodifferentiator3/1(In1)
  pseudodifferentiator3/1(Out1) -> Mux/3
  pseudodifferentiator1/1(Out1) -> Mux/2
  pseudodifferentiator2/1(Out1) -> Mux/1
  In1/1 -> Demux/1
  Mux/1 -> Out1/1

== system simulation_X4_PIDout/Plant model1/2nd order system1/2order ==
  In1 : Inport
  -Gain1 : Gain  Gain=omega_n_m^2
  Gain1 : Gain  Gain=omega_n_m^2
  Gain2 : Gain  Gain=2*xi_m*omega_n_m
  Integrator : Integrator
  Integrator1 : Integrator  InitialCondition=4000
  Scope : Scope
  Scope1 : Scope
  Sum : Sum  Inputs=|+--
  Out1 : Outport
  wires:
  Sum/1 -> Integrator/1
  Integrator/1 -> Integrator1/1, Gain2/1, Scope/1
  Gain2/1 -> Sum/3
  Integrator1/1 -> Scope1/1, -Gain1/1, Out1/1
  Gain1/1 -> Sum/1
  -Gain1/1 -> Sum/2
  In1/1 -> Gain1/1

== system simulation_X4_PIDout/Plant model1/2nd order system1/2order1 ==
  In1 : Inport
  -Gain1 : Gain  Gain=omega_n_m^2
  Gain1 : Gain  Gain=omega_n_m^2
  Gain2 : Gain  Gain=2*xi_m*omega_n_m
  Integrator : Integrator
  Integrator1 : Integrator  InitialCondition=4000
  Scope : Scope
  Scope1 : Scope
  Sum : Sum  Inputs=|+--
  Out1 : Outport
  wires:
  Sum/1 -> Integrator/1
  Integrator/1 -> Integrator1/1, Gain2/1, Scope/1
  Gain2/1 -> Sum/3
  Integrator1/1 -> Scope1/1, -Gain1/1, Out1/1
  Gain1/1 -> Sum/1
  -Gain1/1 -> Sum/2
  In1/1 -> Gain1/1

== system simulation_X4_PIDout/Plant model1/2nd order system1/2order2 ==
  In1 : Inport
  -Gain1 : Gain  Gain=omega_n_m^2
  Gain1 : Gain  Gain=omega_n_m^2
  Gain2 : Gain  Gain=2*xi_m*omega_n_m
  Integrator : Integrator
  Integrator1 : Integrator  InitialCondition=4000
  Scope : Scope
  Scope1 : Scope
  Sum : Sum  Inputs=|+--
  Out1 : Outport
  wires:
  Sum/1 -> Integrator/1
  Integrator/1 -> Integrator1/1, Gain2/1, Scope/1
  Gain2/1 -> Sum/3
  Integrator1/1 -> Scope1/1, -Gain1/1, Out1/1
  Gain1/1 -> Sum/1
  -Gain1/1 -> Sum/2
  In1/1 -> Gain1/1

== system simulation_X4_PIDout/Plant model1/2nd order system1/2order3 ==
  In1 : Inport
  -Gain1 : Gain  Gain=omega_n_m^2
  Gain1 : Gain  Gain=omega_n_m^2
  Gain2 : Gain  Gain=2*xi_m*omega_n_m
  Integrator : Integrator
  Integrator1 : Integrator  InitialCondition=4000
  Scope : Scope
  Scope1 : Scope
  Sum : Sum  Inputs=|+--
  Out1 : Outport
  wires:
  Sum/1 -> Integrator/1
  Integrator/1 -> Integrator1/1, Gain2/1, Scope/1
  Gain2/1 -> Sum/3
  Integrator1/1 -> Scope1/1, -Gain1/1, Out1/1
  Gain1/1 -> Sum/1
  -Gain1/1 -> Sum/2
  In1/1 -> Gain1/1

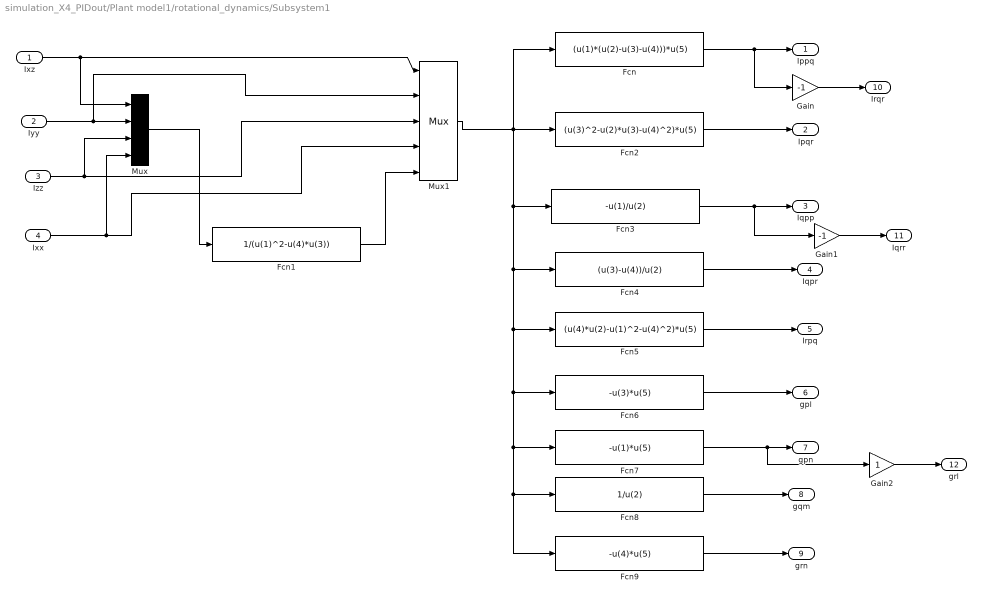
== system simulation_X4_PIDout/Plant model1/rotational_dynamics/Subsystem1 ==
  Ixz : Inport
  Iyy : Inport  Port=2
  Izz : Inport  Port=3
  Ixx : Inport  Port=4
  Fcn : Fcn  Expr=(u(1)*(u(2)-u(3)-u(4)))*u(5)
  Fcn1 : Fcn  Expr=1/(u(1)^2-u(4)*u(3))
  Fcn2 : Fcn  Expr=(u(3)^2-u(2)*u(3)-u(4)^2)*u(5)
  Fcn3 : Fcn  Expr=-u(1)/u(2)
  Fcn4 : Fcn  Expr=(u(3)-u(4))/u(2)
  Fcn5 : Fcn  Expr=(u(4)*u(2)-u(1)^2-u(4)^2)*u(5)
  Fcn6 : Fcn  Expr=-u(3)*u(5)
  Fcn7 : Fcn  Expr=-u(1)*u(5)
  Fcn8 : Fcn  Expr=1/u(2)
  Fcn9 : Fcn  Expr=-u(4)*u(5)
  Gain : Gain  Gain=-1
  Gain1 : Gain  Gain=-1
  Gain2 : Gain
  Mux : Mux
  Mux1 : Mux  Inputs=5
  Ippq : Outport
  Ipqr : Outport  Port=2
  Iqpp : Outport  Port=3
  Iqpr : Outport  Port=4
  Irpq : Outport  Port=5
  gpl : Outport  Port=6
  gpn : Outport  Port=7
  gqm : Outport  Port=8
  grn : Outport  Port=9
  Irqr : Outport  Port=10
  Iqrr : Outport  Port=11
  grl : Outport  Port=12
  wires:
  Ixz/1 -> Mux/1, Mux1/1
  Iyy/1 -> Mux/2, Mux1/2
  Izz/1 -> Mux/3, Mux1/3
  Ixx/1 -> Mux/4, Mux1/4
  Mux/1 -> Fcn1/1
  Fcn1/1 -> Mux1/5
  Fcn/1 -> Ippq/1, Gain/1
  Mux1/1 -> Fcn/1, Fcn2/1, Fcn3/1, Fcn4/1, Fcn5/1, Fcn6/1, Fcn7/1, Fcn8/1, Fcn9/1
  Fcn2/1 -> Ipqr/1
  Fcn3/1 -> Iqpp/1, Gain1/1
  Fcn4/1 -> Iqpr/1
  Fcn5/1 -> Irpq/1
  Fcn6/1 -> gpl/1
  Fcn7/1 -> gpn/1, Gain2/1
  Fcn8/1 -> gqm/1
  Fcn9/1 -> grn/1
  Gain/1 -> Irqr/1
  Gain1/1 -> Iqrr/1
  Gain2/1 -> grl/1

== system simulation_X4_PIDout/altitude control/innner loop controller/Subsystem ==
  In1 : Inport
  Gain1 : Gain  Gain=2*2*4*omega_trans_x_out
  Gain2 : Gain  Gain=(4*omega_trans_x_out)^2
  Integrator : Integrator
  Scope2 : Scope
  Scope3 : Scope
  Scope5 : Scope
  Sum1 : Sum  Inputs=|++
  Out1 : Outport
  wires:
  In1/1 -> Scope3/1, Gain1/1, Scope2/1, Integrator/1
  Gain1/1 -> Sum1/2
  Gain2/1 -> Sum1/1
  Integrator/1 -> Gain2/1, Scope5/1
  Sum1/1 -> Out1/1

== system simulation_X4_PIDout/altitude control/innner loop controller/Subsystem1 ==
  In1 : Inport
  Gain1 : Gain  Gain=2*2*4*omega_trans_y_out
  Gain2 : Gain  Gain=(4*omega_trans_y_out)^2
  Integrator : Integrator
  Scope2 : Scope
  Scope3 : Scope
  Scope5 : Scope
  Sum1 : Sum  Inputs=|++
  Out1 : Outport
  wires:
  In1/1 -> Scope3/1, Gain1/1, Scope2/1, Integrator/1
  Gain1/1 -> Sum1/2
  Gain2/1 -> Sum1/1
  Integrator/1 -> Gain2/1, Scope5/1
  Sum1/1 -> Out1/1

== system simulation_X4_PIDout/altitude control/innner loop controller/Subsystem2 ==
  In1 : Inport
  Gain1 : Gain  Gain=2*2.828*1.5*4*omega_trans_z_out
  Gain2 : Gain  Gain=(4*omega_trans_z_out)^2
  Integrator : Integrator
  Scope2 : Scope
  Scope3 : Scope
  Scope5 : Scope
  Sum1 : Sum  Inputs=|++
  Out1 : Outport
  wires:
  In1/1 -> Scope3/1, Gain1/1, Scope2/1, Integrator/1
  Gain1/1 -> Sum1/2
  Gain2/1 -> Sum1/1
  Integrator/1 -> Gain2/1, Scope5/1
  Sum1/1 -> Out1/1

== system simulation_X4_PIDout/altitude control/outer loop controller/Subsystem ==
  In1 : Inport
  In2 : Inport  Port=2
  Add3 : Sum  Inputs=+++
  Gain1 : Gain  Gain=XP
  Gain2 : Gain  Gain=XI
  Gain3 : Gain  Gain=XD
  Integrator : Integrator
  Out1 : Outport
  wires:
  In1/1 -> Gain1/1, Integrator/1
  Integrator/1 -> Gain2/1
  Gain2/1 -> Add3/1
  Gain1/1 -> Add3/2
  Gain3/1 -> Add3/3
  Add3/1 -> Out1/1
  In2/1 -> Gain3/1

== system simulation_X4_PIDout/altitude control/outer loop controller/Subsystem1 ==
  In1 : Inport
  In2 : Inport  Port=2
  Add3 : Sum  Inputs=+++
  Gain1 : Gain  Gain=YP
  Gain2 : Gain  Gain=YI
  Gain3 : Gain  Gain=YD
  Integrator : Integrator
  Out1 : Outport
  wires:
  In1/1 -> Gain1/1, Integrator/1
  Integrator/1 -> Gain2/1
  Gain2/1 -> Add3/1
  Gain1/1 -> Add3/2
  Gain3/1 -> Add3/3
  Add3/1 -> Out1/1
  In2/1 -> Gain3/1

== system simulation_X4_PIDout/altitude control/outer loop controller/Subsystem2 ==
  In1 : Inport
  In2 : Inport  Port=2
  Add3 : Sum  Inputs=+++
  Gain1 : Gain  Gain=ZP
  Gain2 : Gain  Gain=ZI
  Gain3 : Gain  Gain=ZD
  Integrator : Integrator
  Out1 : Outport
  wires:
  In1/1 -> Gain1/1, Integrator/1
  Integrator/1 -> Gain2/1
  Gain2/1 -> Add3/1
  Gain1/1 -> Add3/2
  Gain3/1 -> Add3/3
  Add3/1 -> Out1/1
  In2/1 -> Gain3/1

== system simulation_X4_PIDout/altitude control/vz pseduo inverter/pseudodifferentiator ==
  In1 : Inport
  Demux : Demux  Outputs=3
  Mux : Mux  Inputs=3
  pseudodifferentiator1 : Subsystem
  pseudodifferentiator2 : Subsystem
  pseudodifferentiator3 : Subsystem
  Out1 : Outport
  wires:
  Demux/1 -> pseudodifferentiator2/1(In1)
  Demux/2 -> pseudodifferentiator1/1(In1)
  Demux/3 -> pseudodifferentiator3/1(In1)
  pseudodifferentiator3/1(Out1) -> Mux/3
  pseudodifferentiator1/1(Out1) -> Mux/2
  pseudodifferentiator2/1(Out1) -> Mux/1
  In1/1 -> Demux/1
  Mux/1 -> Out1/1

== system simulation_X4_PIDout/altitude control/vz pseduo inverter/pseudodifferentiator1 ==
  In1 : Inport
  Demux : Demux  Outputs=3
  Mux : Mux  Inputs=3
  pseudodifferentiator1 : Subsystem
  pseudodifferentiator2 : Subsystem
  pseudodifferentiator3 : Subsystem
  Out1 : Outport
  wires:
  Demux/1 -> pseudodifferentiator2/1(In1)
  Demux/2 -> pseudodifferentiator1/1(In1)
  Demux/3 -> pseudodifferentiator3/1(In1)
  pseudodifferentiator3/1(Out1) -> Mux/3
  pseudodifferentiator1/1(Out1) -> Mux/2
  pseudodifferentiator2/1(Out1) -> Mux/1
  In1/1 -> Demux/1
  Mux/1 -> Out1/1

== system simulation_X4_PIDout/Attitude control/rotational pseduo inverter/pseudodifferentiator/pseudodifferentiator1 ==
  In1 : Inport
  -Gain1 : Gain  Gain=25
  Derivative : Derivative
  Gain1 : Gain  Gain=25
  Gain2 : Gain  Gain=2*5*1.414
  Integrator : Integrator
  Integrator1 : Integrator
  Scope : Scope
  Scope1 : Scope
  Sum : Sum  Inputs=|+--
  Out1 : Outport
  wires:
  Sum/1 -> Integrator/1
  Integrator/1 -> Integrator1/1, Gain2/1, Scope/1
  Gain2/1 -> Sum/3
  Integrator1/1 -> Scope1/1, -Gain1/1, Derivative/1
  Gain1/1 -> Sum/1
  -Gain1/1 -> Sum/2
  In1/1 -> Gain1/1
  Derivative/1 -> Out1/1

== system simulation_X4_PIDout/Attitude control/rotational pseduo inverter/pseudodifferentiator/pseudodifferentiator2 ==
  In1 : Inport
  -Gain1 : Gain  Gain=25
  Derivative : Derivative
  Gain1 : Gain  Gain=25
  Gain2 : Gain  Gain=2*5*1.414
  Integrator : Integrator
  Integrator1 : Integrator
  Scope : Scope
  Scope1 : Scope
  Sum : Sum  Inputs=|+--
  Out1 : Outport
  wires:
  Sum/1 -> Integrator/1
  Integrator/1 -> Integrator1/1, Gain2/1, Scope/1
  Gain2/1 -> Sum/3
  Integrator1/1 -> Scope1/1, -Gain1/1, Derivative/1
  Gain1/1 -> Sum/1
  -Gain1/1 -> Sum/2
  In1/1 -> Gain1/1
  Derivative/1 -> Out1/1

== system simulation_X4_PIDout/Attitude control/rotational pseduo inverter/pseudodifferentiator/pseudodifferentiator3 ==
  In1 : Inport
  -Gain1 : Gain  Gain=25
  Derivative : Derivative
  Gain1 : Gain  Gain=25
  Gain2 : Gain  Gain=2*5*1.414
  Integrator : Integrator
  Integrator1 : Integrator
  Scope : Scope
  Scope1 : Scope
  Sum : Sum  Inputs=|+--
  Out1 : Outport
  wires:
  Sum/1 -> Integrator/1
  Integrator/1 -> Integrator1/1, Gain2/1, Scope/1
  Gain2/1 -> Sum/3
  Integrator1/1 -> Scope1/1, -Gain1/1, Derivative/1
  Gain1/1 -> Sum/1
  -Gain1/1 -> Sum/2
  In1/1 -> Gain1/1
  Derivative/1 -> Out1/1

== system simulation_X4_PIDout/Attitude control/rotational pseduo inverter/pseudodifferentiator1/pseudodifferentiator1 ==
  In1 : Inport
  -Gain1 : Gain  Gain=100
  Derivative : Derivative
  Gain1 : Gain  Gain=100
  Gain2 : Gain  Gain=28.28
  Integrator : Integrator
  Integrator1 : Integrator
  Scope : Scope
  Scope1 : Scope
  Sum : Sum  Inputs=|+--
  Out1 : Outport
  wires:
  Sum/1 -> Integrator/1
  Integrator/1 -> Integrator1/1, Gain2/1, Scope/1
  Gain2/1 -> Sum/3
  Integrator1/1 -> Scope1/1, -Gain1/1, Derivative/1
  Gain1/1 -> Sum/1
  -Gain1/1 -> Sum/2
  In1/1 -> Gain1/1
  Derivative/1 -> Out1/1

== system simulation_X4_PIDout/Attitude control/rotational pseduo inverter/pseudodifferentiator1/pseudodifferentiator2 ==
  In1 : Inport
  -Gain1 : Gain  Gain=100
  Derivative : Derivative
  Gain1 : Gain  Gain=100
  Gain2 : Gain  Gain=28.28
  Integrator : Integrator
  Integrator1 : Integrator
  Scope : Scope
  Scope1 : Scope
  Sum : Sum  Inputs=|+--
  Out1 : Outport
  wires:
  Sum/1 -> Integrator/1
  Integrator/1 -> Integrator1/1, Gain2/1, Scope/1
  Gain2/1 -> Sum/3
  Integrator1/1 -> Scope1/1, -Gain1/1, Derivative/1
  Gain1/1 -> Sum/1
  -Gain1/1 -> Sum/2
  In1/1 -> Gain1/1
  Derivative/1 -> Out1/1

== system simulation_X4_PIDout/Attitude control/rotational pseduo inverter/pseudodifferentiator1/pseudodifferentiator3 ==
  In1 : Inport
  -Gain1 : Gain  Gain=100
  Derivative : Derivative
  Gain1 : Gain  Gain=100
  Gain2 : Gain  Gain=28.28
  Integrator : Integrator
  Integrator1 : Integrator
  Scope : Scope
  Scope1 : Scope
  Sum : Sum  Inputs=|+--
  Out1 : Outport
  wires:
  Sum/1 -> Integrator/1
  Integrator/1 -> Integrator1/1, Gain2/1, Scope/1
  Gain2/1 -> Sum/3
  Integrator1/1 -> Scope1/1, -Gain1/1, Derivative/1
  Gain1/1 -> Sum/1
  -Gain1/1 -> Sum/2
  In1/1 -> Gain1/1
  Derivative/1 -> Out1/1

== system simulation_X4_PIDout/altitude control/vz pseduo inverter/pseudodifferentiator/pseudodifferentiator1 ==
  In1 : Inport
  -Gain1 : Gain  Gain=25
  Derivative : Derivative
  Gain1 : Gain  Gain=25
  Gain2 : Gain  Gain=14.14
  Integrator : Integrator
  Integrator1 : Integrator
  Scope : Scope
  Scope1 : Scope
  Sum : Sum  Inputs=|+--
  Out1 : Outport
  wires:
  Sum/1 -> Integrator/1
  Integrator/1 -> Integrator1/1, Gain2/1, Scope/1
  Gain2/1 -> Sum/3
  Integrator1/1 -> Scope1/1, -Gain1/1, Derivative/1
  Gain1/1 -> Sum/1
  -Gain1/1 -> Sum/2
  In1/1 -> Gain1/1
  Derivative/1 -> Out1/1

== system simulation_X4_PIDout/altitude control/vz pseduo inverter/pseudodifferentiator/pseudodifferentiator2 ==
  In1 : Inport
  -Gain1 : Gain  Gain=25
  Derivative : Derivative
  Gain1 : Gain  Gain=25
  Gain2 : Gain  Gain=14.14
  Integrator : Integrator
  Integrator1 : Integrator
  Scope : Scope
  Scope1 : Scope
  Sum : Sum  Inputs=|+--
  Out1 : Outport
  wires:
  Sum/1 -> Integrator/1
  Integrator/1 -> Integrator1/1, Gain2/1, Scope/1
  Gain2/1 -> Sum/3
  Integrator1/1 -> Scope1/1, -Gain1/1, Derivative/1
  Gain1/1 -> Sum/1
  -Gain1/1 -> Sum/2
  In1/1 -> Gain1/1
  Derivative/1 -> Out1/1

== system simulation_X4_PIDout/altitude control/vz pseduo inverter/pseudodifferentiator/pseudodifferentiator3 ==
  In1 : Inport
  -Gain1 : Gain  Gain=25
  Derivative : Derivative
  Gain1 : Gain  Gain=25
  Gain2 : Gain  Gain=14.14
  Integrator : Integrator
  Integrator1 : Integrator
  Scope : Scope
  Scope1 : Scope
  Sum : Sum  Inputs=|+--
  Out1 : Outport
  wires:
  Sum/1 -> Integrator/1
  Integrator/1 -> Integrator1/1, Gain2/1, Scope/1
  Gain2/1 -> Sum/3
  Integrator1/1 -> Scope1/1, -Gain1/1, Derivative/1
  Gain1/1 -> Sum/1
  -Gain1/1 -> Sum/2
  In1/1 -> Gain1/1
  Derivative/1 -> Out1/1

== system simulation_X4_PIDout/altitude control/vz pseduo inverter/pseudodifferentiator1/pseudodifferentiator1 ==
  In1 : Inport
  -Gain1 : Gain  Gain=25
  Derivative : Derivative
  Gain1 : Gain  Gain=25
  Gain2 : Gain  Gain=14.14
  Integrator : Integrator
  Integrator1 : Integrator
  Scope : Scope
  Scope1 : Scope
  Sum : Sum  Inputs=|+--
  Out1 : Outport
  wires:
  Sum/1 -> Integrator/1
  Integrator/1 -> Integrator1/1, Gain2/1, Scope/1
  Gain2/1 -> Sum/3
  Integrator1/1 -> Scope1/1, -Gain1/1, Derivative/1
  Gain1/1 -> Sum/1
  -Gain1/1 -> Sum/2
  In1/1 -> Gain1/1
  Derivative/1 -> Out1/1

== system simulation_X4_PIDout/altitude control/vz pseduo inverter/pseudodifferentiator1/pseudodifferentiator2 ==
  In1 : Inport
  -Gain1 : Gain  Gain=25
  Derivative : Derivative
  Gain1 : Gain  Gain=25
  Gain2 : Gain  Gain=14.14
  Integrator : Integrator
  Integrator1 : Integrator
  Scope : Scope
  Scope1 : Scope
  Sum : Sum  Inputs=|+--
  Out1 : Outport
  wires:
  Sum/1 -> Integrator/1
  Integrator/1 -> Integrator1/1, Gain2/1, Scope/1
  Gain2/1 -> Sum/3
  Integrator1/1 -> Scope1/1, -Gain1/1, Derivative/1
  Gain1/1 -> Sum/1
  -Gain1/1 -> Sum/2
  In1/1 -> Gain1/1
  Derivative/1 -> Out1/1

== system simulation_X4_PIDout/altitude control/vz pseduo inverter/pseudodifferentiator1/pseudodifferentiator3 ==
  In1 : Inport
  -Gain1 : Gain  Gain=25
  Derivative : Derivative
  Gain1 : Gain  Gain=25
  Gain2 : Gain  Gain=14.14
  Integrator : Integrator
  Integrator1 : Integrator
  Scope : Scope
  Scope1 : Scope
  Sum : Sum  Inputs=|+--
  Out1 : Outport
  wires:
  Sum/1 -> Integrator/1
  Integrator/1 -> Integrator1/1, Gain2/1, Scope/1
  Gain2/1 -> Sum/3
  Integrator1/1 -> Scope1/1, -Gain1/1, Derivative/1
  Gain1/1 -> Sum/1
  -Gain1/1 -> Sum/2
  In1/1 -> Gain1/1
  Derivative/1 -> Out1/1
